simulink model "setupModel"  (R2024b)
settings: Solver=FixedStepAuto  StartTime=0.0  StopTime=10.0  FixedStep=Tsim  RelTol=1e-3
undefined symbols (not defined in the file or in its folder): Do, omega
settings Model: Creator=sung0058  LastModifiedBy=tnoguchi
settings OptimizationCC: DefaultParameterBehavior=Inlined  EnhancedBackFolding=on  PassReuseOutputArgsAs=Individual arguments  ZeroExternalMemoryAtStartup=off  ZeroInternalMemoryAtStartup=off  OptimizeBlockOrder=speed  DifferentSizesBufferReuse=on  OptimizationCustomize=off  EfficientTunableParamExpr=on
settings DebuggingCC: ParameterTunabilityLossMsg=error
settings SFSimCC: MATLABDynamicMemAlloc=off
settings RTWCC: Description=Embedded Coder  SystemTargetFile=ert.tlc  GenCodeOnly=on  TemplateMakefile=ert_default_tmf
settings CodeAppCC: ForceParamTrailComments=on  IgnoreCustomStorageClasses=off  OperatorAnnotations=on  SimulinkDataObjDesc=on  SFDataObjDesc=on  InsertBlockDesc=on
settings ERTTargetCC: TargetLangStandard=C99 (ISO)  ERTCustomFileTemplate=example_file_process.tlc
settings ConfigComp: CovBoundaryAbsTol=1.0e-5

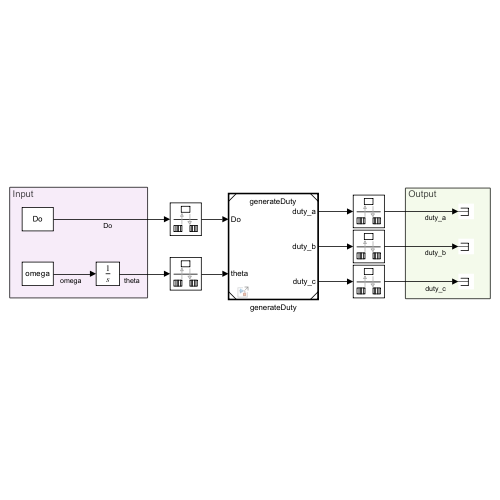
[thumbnail: Simulink's stored preview of the top-level diagram]
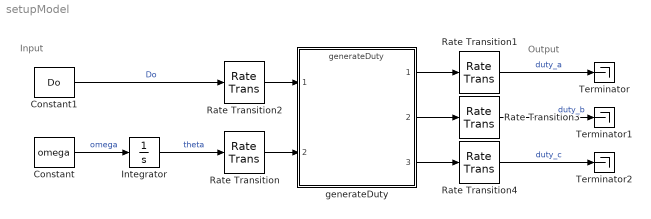
== system setupModel ==
  note: Output
  note: Input
  Constant : Constant  Value=omega
  Constant1 : Constant  Value=Do
  Integrator : Integrator
  Rate Transition : RateTransition  OutPortSampleTime=Ts
  Rate Transition1 : RateTransition
  Rate Transition2 : RateTransition  OutPortSampleTime=Ts
  Rate Transition3 : RateTransition
  Rate Transition4 : RateTransition
  Terminator : Terminator
  Terminator1 : Terminator
  Terminator2 : Terminator
  generateDuty : ModelReference  ModelNameDialog=generateDuty  SimulationMode=Normal  ModelReferenceVersion=1.15
  wires:
  Constant/1 -> Integrator/1  "omega"
  Integrator/1 -> Rate Transition/1  "theta"
  Constant1/1 -> Rate Transition2/1  "Do"
  Rate Transition1/1 -> Terminator/1  "duty_a"
  Rate Transition3/1 -> Terminator1/1  "duty_b"
  Rate Transition4/1 -> Terminator2/1  "duty_c"
  Rate Transition2/1 -> generateDuty/1
  Rate Transition/1 -> generateDuty/2
  generateDuty/1 -> Rate Transition1/1
  generateDuty/2 -> Rate Transition3/1
  generateDuty/3 -> Rate Transition4/1
